simulink library "lib_Convection_FCVertRectCavity"  (R2015a)
settings: Solver=ode45  StartTime=0.0  StopTime=10.0  RelTol=1e-3
libraries: simulink x19, lib_GenTools_MinMax x1
settings Model: Creator=jlkratz  LastModifiedBy=jlkratz

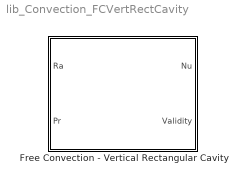
== system lib_Convection_FCVertRectCavity ==
  Free Convection - Vertical Rectangular Cavity : Subsystem  mask(TSAT: Vertical Rectangular Cavity){AR_M=10}
      mask prompts: AR_M "AR_M - Aspect ratio of the rectangular cavity (H/L) where H is the height and L is the distance between the hot and cold walls"
      mask help:
      | This block estimates the average Nusselt number of free convection within a vertical cavity.  The vertical surfaces are heated and cooled while the horizontal surfaces are adiabatic. The flow motion is characterized by a recirculating or cellular flow for which fluid ascends along the hot wall and descends along the cold wall. A set of empirical correlation is employed by this block. Which is active is dependent on the Rayliegh number and aspect ratio (H/L). H is the height of the cavity and L is the distance between the hot and cold surfaces. See the block help menu for the correlations and their restrictions. In For small Rayliegh numbers, Ra <= 1000, the buoyancy-driven flow is weak and, in the absence of radiation, heat transfer is primarily by conduction -> Nu = 1. Note that all fluid properrties should be evaluated at average of the hot and cold surface. Also note that the charateristic length used to calculate the Rayleigh number should be the distance between the hot and cold surfaces (L).
      |
      | See the help menu for more information.
      mask Help: web(which('Convection_TSAT_FCVertRectCavity.html'),'-helpbrowser')

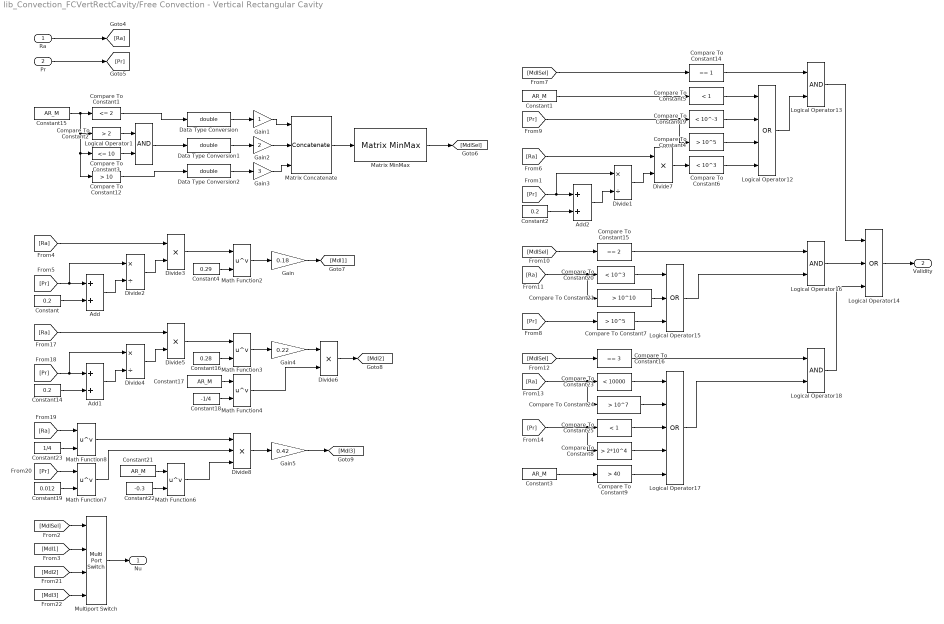
== system lib_Convection_FCVertRectCavity/Free Convection - Vertical Rectangular Cavity ==
  Ra : Inport
  Pr : Inport  Port=2
  Add : Sum
  Add1 : Sum
  Add2 : Sum
  Compare To Constant1 : simulink/Logic and Bit Operations/Compare To Constant  relop=<=  const=2  OutDataTypeStr=boolean
  Compare To Constant12 : simulink/Logic and Bit Operations/Compare To Constant  relop=>  const=10  OutDataTypeStr=boolean
  Compare To Constant14 : simulink/Logic and Bit Operations/Compare To Constant  relop===  const=1  OutDataTypeStr=boolean
  Compare To Constant15 : simulink/Logic and Bit Operations/Compare To Constant  relop===  const=2  OutDataTypeStr=boolean
  Compare To Constant16 : simulink/Logic and Bit Operations/Compare To Constant  relop===  const=3  OutDataTypeStr=boolean
  Compare To Constant19 : simulink/Logic and Bit Operations/Compare To Constant  relop=<  const=10^-3  OutDataTypeStr=boolean
  Compare To Constant2 : simulink/Logic and Bit Operations/Compare To Constant  relop=>  const=2  OutDataTypeStr=boolean
  Compare To Constant20 : simulink/Logic and Bit Operations/Compare To Constant  relop=<  const=10^3  OutDataTypeStr=boolean
  Compare To Constant21 : simulink/Logic and Bit Operations/Compare To Constant  relop=>  const=10^10  OutDataTypeStr=boolean
  Compare To Constant23 : simulink/Logic and Bit Operations/Compare To Constant  relop=<  const=10000  OutDataTypeStr=boolean
  Compare To Constant24 : simulink/Logic and Bit Operations/Compare To Constant  relop=>  const=10^7  OutDataTypeStr=boolean
  Compare To Constant25 : simulink/Logic and Bit Operations/Compare To Constant  relop=<  const=1  OutDataTypeStr=boolean
  Compare To Constant3 : simulink/Logic and Bit Operations/Compare To Constant  relop=<=  const=10  OutDataTypeStr=boolean
  Compare To Constant4 : simulink/Logic and Bit Operations/Compare To Constant  relop=>  const=10^5  OutDataTypeStr=boolean
  Compare To Constant5 : simulink/Logic and Bit Operations/Compare To Constant  relop=<  const=1  OutDataTypeStr=boolean
  Compare To Constant6 : simulink/Logic and Bit Operations/Compare To Constant  relop=<  const=10^3  OutDataTypeStr=boolean
  Compare To Constant7 : simulink/Logic and Bit Operations/Compare To Constant  relop=>  const=10^5  OutDataTypeStr=boolean
  Compare To Constant8 : simulink/Logic and Bit Operations/Compare To Constant  relop=>  const=2*10^4  OutDataTypeStr=boolean
  Compare To Constant9 : simulink/Logic and Bit Operations/Compare To Constant  relop=>  const=40  OutDataTypeStr=boolean
  Constant : Constant  Value=0.2
  Constant{1,3,15,17,21} (5 alike) : Constant  Value=AR_M
  Constant14 : Constant  Value=0.2
  Constant16 : Constant  Value=0.28
  Constant18 : Constant  Value=-1/4
  Constant19 : Constant  Value=0.012
  Constant2 : Constant  Value=0.2
  Constant22 : Constant  Value=-0.3
  Constant23 : Constant  Value=1/4
  Constant4 : Constant  Value=0.29
  Data Type Conversion : DataTypeConversion  OutDataTypeStr=double
  Data Type Conversion1 : DataTypeConversion  OutDataTypeStr=double
  Data Type Conversion2 : DataTypeConversion  OutDataTypeStr=double
  Divide1 : Product  Inputs=*/
  Divide2 : Product  Inputs=*/
  Divide{3,5..7} (4 alike) : Product  Inputs=**
  Divide4 : Product  Inputs=*/
  Divide8 : Product  Inputs=***
  Gain : Gain  Gain=0.18
  Gain1 : Gain
  Gain2 : Gain  Gain=2
  Gain3 : Gain  Gain=3
  Gain4 : Gain  Gain=0.22
  Gain5 : Gain  Gain=0.42
  Logical Operator{1,13,16,18} (4 alike) : Logic  AllPortsSameDT=off  OutDataTypeStr=boolean
  Logical Operator12 : Logic  Operator=OR  Inputs=4  AllPortsSameDT=off  OutDataTypeStr=boolean
  Logical Operator14 : Logic  Operator=OR  Inputs=3  AllPortsSameDT=off  OutDataTypeStr=boolean
  Logical Operator15 : Logic  Operator=OR  Inputs=3  AllPortsSameDT=off  OutDataTypeStr=boolean
  Logical Operator17 : Logic  Operator=OR  Inputs=5  AllPortsSameDT=off  OutDataTypeStr=boolean
  Math Function{2..4,6..8} (6 alike) : Math  Operator=pow  SaturateOnIntegerOverflow=on
  Matrix Concatenate : Concatenate  NumInputs=3  Mode=Multidimensional array  ConcatenateDimension=2
  Matrix MinMax : lib_GenTools_MinMax/Matrix MinMax  rows_M=on  cols_M=off  all_M=off  minmax_M=off  BN_M=gcb
  Multiport Switch : MultiPortSwitch
  Nu : Outport
  Validity : Outport  Port=2
  wires:
  Compare To Constant12/1 -> Data Type Conversion2/1
  Compare To Constant9/1 -> Logical Operator17/5
  Constant3/1 -> Compare To Constant9/1
  Compare To Constant8/1 -> Logical Operator17/4
  Compare To Constant7/1 -> Logical Operator15/3
  [Pr] -> Compare To Constant7/1
  Compare To Constant6/1 -> Logical Operator12/4
  Divide7/1 -> Compare To Constant6/1
  Compare To Constant19/1 -> Logical Operator12/2
  Compare To Constant4/1 -> Logical Operator12/3
  [Ra] -> Divide7/1
  Divide1/1 -> Divide7/2
  Add2/1 -> Divide1/2
  Constant2/1 -> Add2/2
  [Pr] -> Add2/1, Divide1/1
  Compare To Constant5/1 -> Logical Operator12/1
  Constant1/1 -> Compare To Constant5/1
  [Mdl3] -> Multiport Switch/4
  [Mdl2] -> Multiport Switch/3
  [Mdl1] -> Multiport Switch/2
  Multiport Switch/1 -> Nu/1
  Gain5/1 -> [Mdl3]
  Divide8/1 -> Gain5/1
  Math Function6/1 -> Divide8/3
  Math Function7/1 -> Divide8/2
  Math Function8/1 -> Divide8/1
  Constant23/1 -> Math Function8/2
  [Ra] -> Math Function8/1
  Constant19/1 -> Math Function7/2
  [Pr] -> Math Function7/1
  Constant22/1 -> Math Function6/2
  Constant21/1 -> Math Function6/1
  Divide6/1 -> [Mdl2]
  Math Function4/1 -> Divide6/2
  Gain4/1 -> Divide6/1
  Constant18/1 -> Math Function4/2
  Constant17/1 -> Math Function4/1
  Math Function3/1 -> Gain4/1
  Constant16/1 -> Math Function3/2
  Divide5/1 -> Math Function3/1
  Divide4/1 -> Divide5/2
  [Ra] -> Divide5/1
  Add1/1 -> Divide4/2
  Constant14/1 -> Add1/2
  [Pr] -> Divide4/1, Add1/1
  Gain/1 -> [Mdl1]
  Compare To Constant1/1 -> Data Type Conversion/1
  Logical Operator1/1 -> Data Type Conversion1/1
  Compare To Constant3/1 -> Logical Operator1/2
  Compare To Constant2/1 -> Logical Operator1/1
  Constant15/1 -> Compare To Constant1/1, Compare To Constant12/1, Compare To Constant3/1, Compare To Constant2/1
  Matrix Concatenate/1 -> Matrix MinMax/1
  Gain3/1 -> Matrix Concatenate/3
  Gain2/1 -> Matrix Concatenate/2
  Gain1/1 -> Matrix Concatenate/1
  Data Type Conversion/1 -> Gain1/1
  Data Type Conversion1/1 -> Gain2/1
  Data Type Conversion2/1 -> Gain3/1
  Matrix MinMax/1 -> [MdlSel]
  Math Function2/1 -> Gain/1
  Constant4/1 -> Math Function2/2
  Divide3/1 -> Math Function2/1
  Divide2/1 -> Divide3/2
  [Ra] -> Divide3/1
  Add/1 -> Divide2/2
  Constant/1 -> Add/2
  [Pr] -> Add/1, Divide2/1
  Logical Operator18/1 -> Logical Operator14/3
  Logical Operator16/1 -> Logical Operator14/2
  Logical Operator13/1 -> Logical Operator14/1
  Logical Operator17/1 -> Logical Operator18/2
  Compare To Constant16/1 -> Logical Operator18/1
  Compare To Constant25/1 -> Logical Operator17/3
  Compare To Constant24/1 -> Logical Operator17/2
  Compare To Constant23/1 -> Logical Operator17/1
  [Pr] -> Compare To Constant25/1, Compare To Constant8/1
  [Ra] -> Compare To Constant24/1, Compare To Constant23/1
  [MdlSel] -> Compare To Constant16/1
  Logical Operator15/1 -> Logical Operator16/2
  Compare To Constant15/1 -> Logical Operator16/1
  Compare To Constant21/1 -> Logical Operator15/2
  Compare To Constant20/1 -> Logical Operator15/1
  [Ra] -> Compare To Constant21/1, Compare To Constant20/1
  [MdlSel] -> Compare To Constant15/1
  Logical Operator12/1 -> Logical Operator13/2
  Compare To Constant14/1 -> Logical Operator13/1
  [Pr] -> Compare To Constant19/1, Compare To Constant4/1
  [MdlSel] -> Compare To Constant14/1
  Pr/1 -> [Pr]
  [MdlSel] -> Multiport Switch/1
  Logical Operator14/1 -> Validity/1
  Ra/1 -> [Ra]
